simulink model "ThermalConfirm"  (R2016a)
settings: Solver=FixedStepAuto  StartTime=0.0  StopTime=45*9  FixedStep=500e-6  RelTol=1e-3
libraries: powerlib x94
settings Model: Creator=Patrick  LastModifiedBy=Patrick

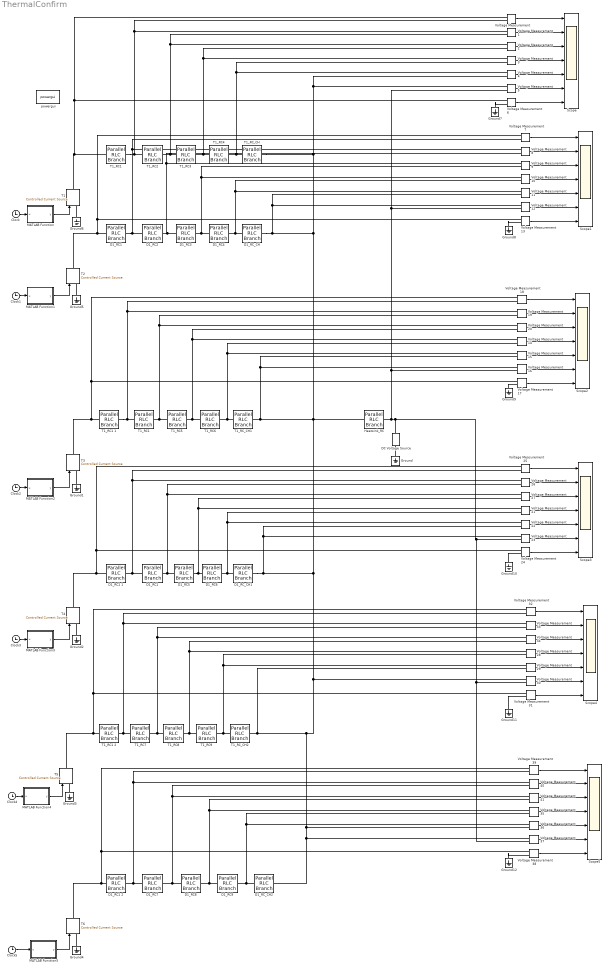
== system ThermalConfirm ==
  Clock{,1..5} (6 alike) : Clock
  D1_RC1 : powerlib/Elements/Parallel RLC Branch  LConnTagsString=a  RConnTagsString=__new0  BranchType=RC  Resistance=0.0526  Inductance=1e-3  SetiL0=off  InitialCurrent=0  Capacitance=0.029/0.0526  Setx0=off  InitialVoltage=0  Measurements=None
  "D1_RC1 " : powerlib/Elements/Parallel RLC Branch  LConnTagsString=a  RConnTagsString=__new0  BranchType=RC  Resistance=0.0081  Inductance=1e-3  SetiL0=off  InitialCurrent=0  Capacitance=0.00088/0.0081  Setx0=off  InitialVoltage=0  Measurements=None
  D1_RC1 1 : powerlib/Elements/Parallel RLC Branch  LConnTagsString=a  RConnTagsString=__new0  BranchType=RC  Resistance=0.0081  Inductance=1e-3  SetiL0=off  InitialCurrent=0  Capacitance=0.00088/0.0081  Setx0=off  InitialVoltage=0  Measurements=None
  D1_RC1 2 : powerlib/Elements/Parallel RLC Branch  LConnTagsString=a  RConnTagsString=__new0  BranchType=RC  Resistance=0.0081  Inductance=1e-3  SetiL0=off  InitialCurrent=0  Capacitance=0.00088/0.0081  Setx0=off  InitialVoltage=0  Measurements=None
  D1_RC2 : powerlib/Elements/Parallel RLC Branch  LConnTagsString=a  RConnTagsString=__new0  BranchType=RC  Resistance=0.0526  Inductance=1e-3  SetiL0=off  InitialCurrent=0  Capacitance=0.029/0.0526  Setx0=off  InitialVoltage=0  Measurements=None
  D1_RC3 : powerlib/Elements/Parallel RLC Branch  LConnTagsString=a  RConnTagsString=__new0  BranchType=RC  Resistance=0.00697  Inductance=1e-3  SetiL0=off  InitialCurrent=0  Capacitance=0.17225/0.00697  Setx0=off  InitialVoltage=0  Measurements=None
  D1_RC4 : powerlib/Elements/Parallel RLC Branch  LConnTagsString=a  RConnTagsString=__new0  BranchType=RC  Resistance=0.00531  Inductance=1e-3  SetiL0=off  InitialCurrent=0  Capacitance=5.18101/0.00531  Setx0=off  InitialVoltage=0  Measurements=None
  D1_RC5 : powerlib/Elements/Parallel RLC Branch  LConnTagsString=a  RConnTagsString=__new0  BranchType=RC  Resistance=0.00697  Inductance=1e-3  SetiL0=off  InitialCurrent=0  Capacitance=0.17225/0.00697  Setx0=off  InitialVoltage=0  Measurements=None
  D1_RC6 : powerlib/Elements/Parallel RLC Branch  LConnTagsString=a  RConnTagsString=__new0  BranchType=RC  Resistance=0.00531  Inductance=1e-3  SetiL0=off  InitialCurrent=0  Capacitance=5.18101/0.00531  Setx0=off  InitialVoltage=0  Measurements=None
  D1_RC7 : powerlib/Elements/Parallel RLC Branch  LConnTagsString=a  RConnTagsString=__new0  BranchType=RC  Resistance=0.0526  Inductance=1e-3  SetiL0=off  InitialCurrent=0  Capacitance=0.029/0.0526  Setx0=off  InitialVoltage=0  Measurements=None
  D1_RC8 : powerlib/Elements/Parallel RLC Branch  LConnTagsString=a  RConnTagsString=__new0  BranchType=RC  Resistance=0.00697  Inductance=1e-3  SetiL0=off  InitialCurrent=0  Capacitance=0.17225/0.00697  Setx0=off  InitialVoltage=0  Measurements=None
  D1_RC9 : powerlib/Elements/Parallel RLC Branch  LConnTagsString=a  RConnTagsString=__new0  BranchType=RC  Resistance=0.00531  Inductance=1e-3  SetiL0=off  InitialCurrent=0  Capacitance=5.18101/0.00531  Setx0=off  InitialVoltage=0  Measurements=None
  D1_RC_CH : powerlib/Elements/Parallel RLC Branch  LConnTagsString=a  RConnTagsString=__new0  BranchType=RC  Resistance=0.0378  Inductance=1e-3  SetiL0=off  InitialCurrent=0  Capacitance=5/0.0378  Setx0=off  InitialVoltage=0  Measurements=None
  D1_RC_CH1 : powerlib/Elements/Parallel RLC Branch  LConnTagsString=a  RConnTagsString=__new0  BranchType=RC  Resistance=0.0378  Inductance=1e-3  SetiL0=off  InitialCurrent=0  Capacitance=5/0.0378  Setx0=off  InitialVoltage=0  Measurements=None
  D1_RC_CH2 : powerlib/Elements/Parallel RLC Branch  LConnTagsString=a  RConnTagsString=__new0  BranchType=RC  Resistance=0.0378  Inductance=1e-3  SetiL0=off  InitialCurrent=0  Capacitance=5/0.0378  Setx0=off  InitialVoltage=0  Measurements=None
  DC Voltage Source : powerlib/Electrical Sources/DC Voltage Source  Amplitude=35  Measurements=None
  Ground{,1..12} (13 alike) : powerlib/Elements/Ground  LConnTagsString=a
  Heatsink_RC : powerlib/Elements/Parallel RLC Branch  LConnTagsString=a  RConnTagsString=__new0  BranchType=RC  Resistance=0.12  Inductance=1e-3  SetiL0=off  InitialCurrent=0  Capacitance=45/0.12  Setx0=off  InitialVoltage=0  Measurements=None
  MATLAB Function : MATLAB Function  TreatAsAtomicUnit=on
  MATLAB Function1 : MATLAB Function  TreatAsAtomicUnit=on
  MATLAB Function2 : MATLAB Function  TreatAsAtomicUnit=on
  MATLAB Function3 : MATLAB Function  TreatAsAtomicUnit=on
  MATLAB Function4 : MATLAB Function  TreatAsAtomicUnit=on
  MATLAB Function5 : MATLAB Function  TreatAsAtomicUnit=on
  Scope{,1..5} (6 alike) : Scope  NumInputPorts=7
  T{1..6} (6 alike) : powerlib/Electrical Sources/Controlled Current Source  Initialize=on  Source_Type=AC  Amplitude=0  Phase=0  Frequency=0  Measurements=None
  T1_RC1 : powerlib/Elements/Parallel RLC Branch  LConnTagsString=a  RConnTagsString=__new0  BranchType=RC  Resistance=0.00225  Inductance=1e-3  SetiL0=off  InitialCurrent=0  Capacitance=0.00324  Setx0=off  InitialVoltage=0  Measurements=None
  "T1_RC1 " : powerlib/Elements/Parallel RLC Branch  LConnTagsString=a  RConnTagsString=__new0  BranchType=RC  Resistance=0.0017  Inductance=1e-3  SetiL0=off  InitialCurrent=0  Capacitance=0.00053/0.0017  Setx0=off  InitialVoltage=0  Measurements=None
  T1_RC1 1 : powerlib/Elements/Parallel RLC Branch  LConnTagsString=a  RConnTagsString=__new0  BranchType=RC  Resistance=0.0017  Inductance=1e-3  SetiL0=off  InitialCurrent=0  Capacitance=0.00053/0.0017  Setx0=off  InitialVoltage=0  Measurements=None
  T1_RC1 2 : powerlib/Elements/Parallel RLC Branch  LConnTagsString=a  RConnTagsString=__new0  BranchType=RC  Resistance=0.0017  Inductance=1e-3  SetiL0=off  InitialCurrent=0  Capacitance=0.00053/0.0017  Setx0=off  InitialVoltage=0  Measurements=None
  T1_RC2 : powerlib/Elements/Parallel RLC Branch  LConnTagsString=a  RConnTagsString=__new0  BranchType=RC  Resistance=0.00225  Inductance=1e-3  SetiL0=off  InitialCurrent=0  Capacitance=0.00324  Setx0=off  InitialVoltage=0  Measurements=None
  T1_RC3 : powerlib/Elements/Parallel RLC Branch  LConnTagsString=a  RConnTagsString=__new0  BranchType=RC  Resistance=0.03078  Inductance=1e-3  SetiL0=off  InitialCurrent=0  Capacitance=0.03234/0.03078  Setx0=off  InitialVoltage=0  Measurements=None
  T1_RC4 : powerlib/Elements/Parallel RLC Branch  LConnTagsString=a  RConnTagsString=__new0  BranchType=RC  Resistance=0.00216  Inductance=1e-3  SetiL0=off  InitialCurrent=0  Capacitance=8.13887/0.00216  Setx0=off  InitialVoltage=0  Measurements=None
  T1_RC5 : powerlib/Elements/Parallel RLC Branch  LConnTagsString=a  RConnTagsString=__new0  BranchType=RC  Resistance=0.03078  Inductance=1e-3  SetiL0=off  InitialCurrent=0  Capacitance=0.03234/0.03078  Setx0=off  InitialVoltage=0  Measurements=None
  T1_RC6 : powerlib/Elements/Parallel RLC Branch  LConnTagsString=a  RConnTagsString=__new0  BranchType=RC  Resistance=0.00216  Inductance=1e-3  SetiL0=off  InitialCurrent=0  Capacitance=8.13887/0.00216  Setx0=off  InitialVoltage=0  Measurements=None
  T1_RC7 : powerlib/Elements/Parallel RLC Branch  LConnTagsString=a  RConnTagsString=__new0  BranchType=RC  Resistance=0.00225  Inductance=1e-3  SetiL0=off  InitialCurrent=0  Capacitance=0.00324  Setx0=off  InitialVoltage=0  Measurements=None
  T1_RC8 : powerlib/Elements/Parallel RLC Branch  LConnTagsString=a  RConnTagsString=__new0  BranchType=RC  Resistance=0.03078  Inductance=1e-3  SetiL0=off  InitialCurrent=0  Capacitance=0.03234/0.03078  Setx0=off  InitialVoltage=0  Measurements=None
  T1_RC9 : powerlib/Elements/Parallel RLC Branch  LConnTagsString=a  RConnTagsString=__new0  BranchType=RC  Resistance=0.00216  Inductance=1e-3  SetiL0=off  InitialCurrent=0  Capacitance=8.13887/0.00216  Setx0=off  InitialVoltage=0  Measurements=None
  T1_RC_CH : powerlib/Elements/Parallel RLC Branch  LConnTagsString=a  RConnTagsString=__new0  BranchType=RC  Resistance=0.0328  Inductance=1e-3  SetiL0=off  InitialCurrent=0  Capacitance=5/0.0328  Setx0=off  InitialVoltage=0  Measurements=None
  T1_RC_CH1 : powerlib/Elements/Parallel RLC Branch  LConnTagsString=a  RConnTagsString=__new0  BranchType=RC  Resistance=0.0328  Inductance=1e-3  SetiL0=off  InitialCurrent=0  Capacitance=5/0.0328  Setx0=off  InitialVoltage=0  Measurements=None
  T1_RC_CH2 : powerlib/Elements/Parallel RLC Branch  LConnTagsString=a  RConnTagsString=__new0  BranchType=RC  Resistance=0.0328  Inductance=1e-3  SetiL0=off  InitialCurrent=0  Capacitance=5/0.0328  Setx0=off  InitialVoltage=0  Measurements=None
  Voltage Measurement{,1..41} (42 alike) : powerlib/Measurements/Voltage Measurement  PhasorSimulation=off  OutputType=Complex  PSBequivalent=0
  powergui : powerlib/powergui  Priority=1  SimulationMode=Discrete  SolverType=Tustin/Backward Euler (TBE)  SampleTime=500e-6  frequency=60  SPID=off  DisableSnubberDevices=off  DisableRonSwitches=off  DisableVfSwitches=off  SwTol=0  DisplayEquations=off  Interpol=off  ExternalGateDelay=off  methode=off  Ts=10  FunctionMessages=off  echomessages=off  HookPort=off  EnableUseOfTLC=off  x0status=blocks  frequencyindice=0  Pbase=100e6  ErrMax=1e-4  Iterations=50  UnitsV=kV  UnitsW=MW  buscounter=0  RestoreLinks=warning  ResistiveCurrentMeasurement=off  Frange=[0:2:500]  Ylog=off  Xlog=on  ShowGrid=off  save=off  variable=ZData  structure=0  ZoomFFT=off  StartTime=0.0  cycles=1  DisplayStyle=1  fundamental=60  FreqAxis=off  MaxFrequency=1000  frequencyindicesteady=1  RmsSteady=1  display=off
  wires:
  MATLAB Function/1(y) -> T1/1
  Clock/1 -> MATLAB Function/1(u)
  Clock1/1 -> MATLAB Function1/1(u)
  MATLAB Function1/1(y) -> T2/1
  Clock2/1 -> MATLAB Function2/1(u)
  MATLAB Function2/1(y) -> T3/1
  Clock3/1 -> MATLAB Function3/1(u)
  MATLAB Function3/1(y) -> T4/1
  Clock4/1 -> MATLAB Function4/1(u)
  MATLAB Function4/1(y) -> T5/1
  Clock5/1 -> MATLAB Function5/1(u)
  MATLAB Function5/1(y) -> T6/1
  Voltage Measurement/1 -> Scope/1
  Voltage Measurement1/1 -> Scope/2
  Voltage Measurement2/1 -> Scope/3
  Voltage Measurement3/1 -> Scope/4
  Voltage Measurement4/1 -> Scope/5
  Voltage Measurement5/1 -> Scope/6
  Voltage Measurement6/1 -> Scope/7
  Voltage Measurement7/1 -> Scope1/1
  Voltage Measurement8/1 -> Scope1/2
  Voltage Measurement9/1 -> Scope1/3
  Voltage Measurement10/1 -> Scope1/4
  Voltage Measurement11/1 -> Scope1/5
  Voltage Measurement12/1 -> Scope1/6
  Voltage Measurement13/1 -> Scope1/7
  Voltage Measurement18/1 -> Scope2/1
  Voltage Measurement19/1 -> Scope2/2
  Voltage Measurement20/1 -> Scope2/3
  Voltage Measurement14/1 -> Scope2/4
  Voltage Measurement15/1 -> Scope2/5
  Voltage Measurement16/1 -> Scope2/6
  Voltage Measurement17/1 -> Scope2/7
  Voltage Measurement25/1 -> Scope3/1
  Voltage Measurement26/1 -> Scope3/2
  Voltage Measurement27/1 -> Scope3/3
  Voltage Measurement21/1 -> Scope3/4
  Voltage Measurement22/1 -> Scope3/5
  Voltage Measurement23/1 -> Scope3/6
  Voltage Measurement24/1 -> Scope3/7
  Voltage Measurement32/1 -> Scope4/1
  Voltage Measurement33/1 -> Scope4/2
  Voltage Measurement34/1 -> Scope4/3
  Voltage Measurement28/1 -> Scope4/4
  Voltage Measurement29/1 -> Scope4/5
  Voltage Measurement30/1 -> Scope4/6
  Voltage Measurement31/1 -> Scope4/7
  Voltage Measurement39/1 -> Scope5/1
  Voltage Measurement40/1 -> Scope5/2
  Voltage Measurement41/1 -> Scope5/3
  Voltage Measurement35/1 -> Scope5/4
  Voltage Measurement36/1 -> Scope5/5
  Voltage Measurement37/1 -> Scope5/6
  Voltage Measurement38/1 -> Scope5/7
  connections:
  T1/RConn1 -- Voltage Measurement/LConn1 -- Voltage Measurement6/LConn1 -- "T1_RC1 "/LConn1
  T1_RC3/LConn1 -- Voltage Measurement2/LConn1 -- Voltage Measurement1/LConn2 -- T1_RC2/RConn1
  T1_RC4/LConn1 -- Voltage Measurement3/LConn1 -- Voltage Measurement2/LConn2 -- T1_RC3/RConn1
  T1_RC_CH/LConn1 -- Voltage Measurement4/LConn1 -- Voltage Measurement3/LConn2 -- T1_RC4/RConn1
  "T1_RC1 "/RConn1 -- Voltage Measurement1/LConn1 -- Voltage Measurement/LConn2 -- T1_RC2/LConn1
  D1_RC_CH/LConn1 -- Voltage Measurement11/LConn1 -- Voltage Measurement10/LConn2 -- D1_RC4/RConn1
  "D1_RC1 "/RConn1 -- Voltage Measurement7/LConn2 -- Voltage Measurement8/LConn1 -- D1_RC2/LConn1
  T2/RConn1 -- Voltage Measurement7/LConn1 -- Voltage Measurement13/LConn1 -- "D1_RC1 "/LConn1
  D1_RC3/LConn1 -- Voltage Measurement8/LConn2 -- Voltage Measurement9/LConn1 -- D1_RC2/RConn1
  D1_RC4/LConn1 -- Voltage Measurement10/LConn1 -- Voltage Measurement9/LConn2 -- D1_RC3/RConn1
  D1_RC5/LConn1 -- Voltage Measurement27/LConn1 -- Voltage Measurement26/LConn2 -- D1_RC1/RConn1
  T1_RC1 1/LConn1 -- Voltage Measurement17/LConn1 -- Voltage Measurement18/LConn1 -- T3/RConn1
  D1_RC1/LConn1 -- Voltage Measurement26/LConn1 -- Voltage Measurement25/LConn2 -- D1_RC1 1/RConn1
  D1_RC1 1/LConn1 -- Voltage Measurement24/LConn1 -- Voltage Measurement25/LConn1 -- T4/RConn1
  T6/RConn1 -- Voltage Measurement38/LConn1 -- Voltage Measurement39/LConn1 -- D1_RC1 2/LConn1
  T1_RC1 2/LConn1 -- Voltage Measurement31/LConn1 -- Voltage Measurement32/LConn1 -- T5/RConn1
  T1_RC_CH/RConn1 -- Voltage Measurement4/LConn2 -- Voltage Measurement5/LConn1 -- Voltage Measurement12/LConn1 -- Voltage Measurement11/LConn2 -- D1_RC_CH/RConn1 -- Heatsink_RC/LConn1 -- Voltage Measurement30/LConn1 -- Voltage Measurement29/LConn2 -- T1_RC_CH2/RConn1 -- Voltage Measurement36/LConn2 -- D1_RC_CH2/RConn1 -- Voltage Measurement37/LConn1 -- Voltage Measurement23/LConn1 -- Voltage Measurement22/LConn2 -- D1_RC_CH1/RConn1 -- Voltage Measurement16/LConn1 -- Voltage Measurement15/LConn2 -- T1_RC_CH1/RConn1
  DC Voltage Source/RConn1 -- Voltage Measurement37/LConn2 -- Voltage Measurement30/LConn2 -- Voltage Measurement23/LConn2 -- Voltage Measurement16/LConn2 -- Voltage Measurement12/LConn2 -- Voltage Measurement5/LConn2 -- Heatsink_RC/RConn1
  Ground/LConn1 -- DC Voltage Source/LConn1
  Ground1/LConn1 -- T3/LConn1
  Ground2/LConn1 -- T4/LConn1
  Ground3/LConn1 -- T5/LConn1
  Ground4/LConn1 -- T6/LConn1
  D1_RC6/LConn1 -- Voltage Measurement21/LConn1 -- Voltage Measurement27/LConn2 -- D1_RC5/RConn1
  D1_RC_CH1/LConn1 -- Voltage Measurement21/LConn2 -- Voltage Measurement22/LConn1 -- D1_RC6/RConn1
  T1_RC_CH1/LConn1 -- Voltage Measurement15/LConn1 -- Voltage Measurement14/LConn2 -- T1_RC6/RConn1
  T1_RC6/LConn1 -- Voltage Measurement14/LConn1 -- Voltage Measurement20/LConn2 -- T1_RC5/RConn1
  T1_RC5/LConn1 -- Voltage Measurement20/LConn1 -- Voltage Measurement19/LConn2 -- T1_RC1/RConn1
  T1_RC1 1/RConn1 -- Voltage Measurement19/LConn1 -- Voltage Measurement18/LConn2 -- T1_RC1/LConn1
  D1_RC7/LConn1 -- Voltage Measurement40/LConn1 -- Voltage Measurement39/LConn2 -- D1_RC1 2/RConn1
  D1_RC8/LConn1 -- Voltage Measurement41/LConn1 -- Voltage Measurement40/LConn2 -- D1_RC7/RConn1
  D1_RC9/LConn1 -- Voltage Measurement35/LConn1 -- Voltage Measurement41/LConn2 -- D1_RC8/RConn1
  D1_RC_CH2/LConn1 -- Voltage Measurement36/LConn1 -- Voltage Measurement35/LConn2 -- D1_RC9/RConn1
  T1_RC1 2/RConn1 -- Voltage Measurement33/LConn1 -- Voltage Measurement32/LConn2 -- T1_RC7/LConn1
  T1_RC_CH2/LConn1 -- Voltage Measurement29/LConn1 -- Voltage Measurement28/LConn2 -- T1_RC9/RConn1
  T1_RC8/LConn1 -- Voltage Measurement34/LConn1 -- Voltage Measurement33/LConn2 -- T1_RC7/RConn1
  T1_RC9/LConn1 -- Voltage Measurement28/LConn1 -- Voltage Measurement34/LConn2 -- T1_RC8/RConn1
  Ground5/LConn1 -- T2/LConn1
  Ground6/LConn1 -- T1/LConn1
  Ground7/LConn1 -- Voltage Measurement6/LConn2
  Ground8/LConn1 -- Voltage Measurement13/LConn2
  Voltage Measurement17/LConn2 -- Ground9/LConn1
  Ground10/LConn1 -- Voltage Measurement24/LConn2
  Ground11/LConn1 -- Voltage Measurement31/LConn2
  Ground12/LConn1 -- Voltage Measurement38/LConn2

== matlab function ThermalConfirm/MATLAB Function1 ==
  data: u input; y output
function y = fcn(u)
%#codegen
pLossT1 = 100*pi*sin(2*pi*6*u+pi);
if(pLossT1<0)
    out = 0;
else
    out = pLossT1;
end
y = out;

== matlab function ThermalConfirm/MATLAB Function ==
  data: u input; y output
function y = fcn(u)
%#codegen
pLossT1 = 250*pi*sin(2*pi*6*u);
if(pLossT1<0)
    out = 0;
else
    out = pLossT1;
end
y = out;

== matlab function ThermalConfirm/MATLAB Function2 ==
  data: u input; y output
function y = fcn(u)
%#codegen
pLossT1 = 150*pi*sin(2*pi*6*u);
if(pLossT1<0)
    out = 0;
else
    out = pLossT1;
end
y = out;

== matlab function ThermalConfirm/MATLAB Function3 ==
  data: u input; y output
function y = fcn(u)
%#codegen
pLossT1 = 50*pi*sin(2*pi*6*u+pi);
if(pLossT1<0)
    out = 0;
else
    out = pLossT1;
end
y = out;

== matlab function ThermalConfirm/MATLAB Function4 ==
  data: u input; y output
function y = fcn(u)
%#codegen
pLossT1 = 200*pi*sin(2*pi*6*u+pi);
if(pLossT1<0)
    out = 0;
else
    out = pLossT1;
end
y = out;

== matlab function ThermalConfirm/MATLAB Function5 ==
  data: u input; y output
function y = fcn(u)
%#codegen
pLossT1 = 25*pi*sin(2*pi*6*u+pi);
if(pLossT1<0)
    out = 0;
else
    out = pLossT1;
end
y = out;
